simulink model "hcm_bicycle"  (R2017b)
settings: Solver=FixedStepAuto  StartTime=0.0  StopTime=10.0  RelTol=1e-3
values from neighbouring files (symbols this model uses):
  front_rear = 0    [init.m]
  setV = 0    [init.m]
  your_dut = 18    [init.m]
undefined symbols (not defined in the file or in its folder): hcm, sigbuilder_block, Zs0, Zu0
libraries: simulink x1
settings Model: Creator=rvorster  LastModifiedBy=rvorster

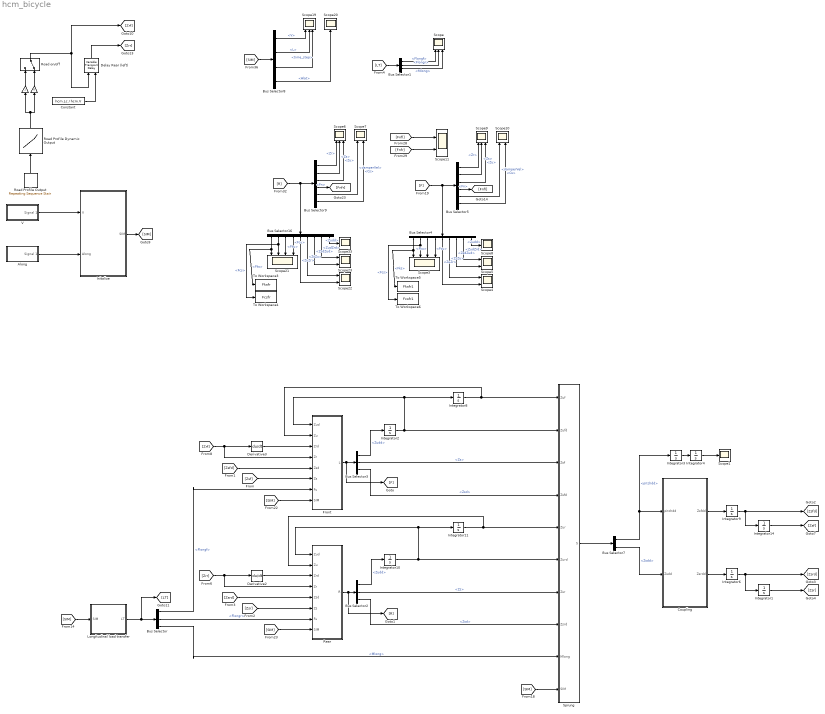
== system hcm_bicycle ==
  " " : Gain
  " " : Gain  Gain=0
  Along : Subsystem  Tag=STV Subsys  LoadFcn=sigbuilder_block('load');  StartFcn=sigbuilder_block('start');  StopFcn=sigbuilder_block('stop');  ClipboardFcn=sigbuilder_block('clipboard');  mask(Sigbuilder block){tuvar=[0:10]}
      mask help: Simulink:masks:SigbuilderBlock_MD
      mask init:
      | if ~strcmp(get_param(bdroot(gcbh),'SimulationStatus'),'stopped') tuvar = sigbuilder_block('maskInit'); end
      settings: CopyFcn=sigbuilder_block('copy');  DeleteFcn=sigbuilder_block('delete');  ModelCloseFcn=sigbuilder_block('modelClose');  PreSaveFcn=sigbuilder_block('preSave');  PauseFcn=sigbuilder_block('pause');  ContinueFcn=sigbuilder_block('continue');  NameChangeFcn=sigbuilder_block('namechange');  OpenFcn=sigbuilder_block('open',[429.75 192 565.5 402.75 ]);  CloseFcn=sigbuilder_block('close');
      mask Display: plot(0, 0, 100, 100,[2, 2, 32, 32, 2], [68, 8, 8, 68, 68],[32, 2], [38, 38], [32, 19, 2],[53, 60, 44], [32, 17, 17, 2],[16, 16, 31, 31]);txt = getActiveGroup(gcbh);text(2, 100, txt,'verticalAlignment', 'top');
  Bus Selector : BusSelector  OutputSignals=Flongf,Flongr,Mlong
  Bus Selector1 : BusSelector  OutputSignals=Flongf,Flongr,Mlong
  Bus Selector16 : BusSelector  OutputSignals=Fks,Fcs,Fku,Fcu,ZuZr,ZsZu,ZsdZud,ZudZrd,Zudd
  Bus Selector2 : BusSelector  OutputSignals=Zudd,Zs,Zsd
  Bus Selector3 : BusSelector  OutputSignals=Zudd,Zs,Zsd
  Bus Selector4 : BusSelector  OutputSignals=Fks,Fcs,Fku,Fcu,ZuZr,ZsZu,ZsdZud,ZudZrd,Zudd
  Bus Selector5 : BusSelector  OutputSignals=Zr,Zs,Zu,Fn,damperVel,Cs
  Bus Selector7 : BusSelector  OutputSignals=pitchdd,Zsdd
  Bus Selector8 : BusSelector  OutputSignals=V,L,time_step,Alat
  Bus Selector9 : BusSelector  OutputSignals=Zr,Zs,Zu,Fn,damperVel,Cs
  Constant : Constant  Value=hcm.Lc / hcm.V
  Coupling : MATLAB Function  TreatAsAtomicUnit=on
  Delay Rear (left) : VariableTransportDelay  VariableDelayType=Variable transport delay  MaximumDelay=10  MaximumPoints=4096
  Derivative2 : Derivative
  Derivative3 : Derivative
  Front : MATLAB Function  TreatAsAtomicUnit=on
  Initalize : MATLAB Function  TreatAsAtomicUnit=on
  Integrator1 : Integrator  InitialCondition=-Zs0(3)
  Integrator{2..4,6,9..10} (6 alike) : Integrator
  Integrator11 : Integrator  InitialCondition=-Zu0(3)
  Integrator14 : Integrator  InitialCondition=-Zs0(1)
  Integrator8 : Integrator  InitialCondition=-Zu0(1)
  Longitudinal load transfer : MATLAB Function  TreatAsAtomicUnit=on
  Rear : MATLAB Function  TreatAsAtomicUnit=on
  Road Profile Dynamic Output : Lookup_n-D  NumberOfTableDimensions=1  BreakpointsForDimension1=[-5:5]  Table=tanh([-5:5])  InternalRulePriority=Speed  RndMeth=Simplest  InputSameDT=on
  Road Profile Output : simulink/Sources/Repeating Sequence Stair  OutValues=hx_left  tsamp=time_step  OutMin=[]  OutMax=[]  OutDataTypeStr=double  OutputDataTypeScalingMode=double  OutDataType=fixdt(0,8)  ConRadixGroup=Best Precision: Vector-wise  OutScaling=2^-12
  "Road on/off " : ManualSwitch  CurrentSetting=0
  Scope{,6,9,19} (4 alike) : Scope  NumInputPorts=3
  Scope{1,8,20,33} (4 alike) : Scope
  Scope{4..5,7,10..11,22..23} (7 alike) : Scope  NumInputPorts=2
  Scope21 : Scope  NumInputPorts=4
  Scope3 : Scope  NumInputPorts=4
  Sprung : MATLAB Function  TreatAsAtomicUnit=on
  To Workspace3 : ToWorkspace  VariableName=Fksfr  SaveFormat=Timeseries  SampleTime=-1
  To Workspace4 : ToWorkspace  VariableName=Fcsfr  SaveFormat=Timeseries  SampleTime=-1
  To Workspace5 : ToWorkspace  VariableName=Fksfr1  SaveFormat=Timeseries  SampleTime=-1
  To Workspace6 : ToWorkspace  VariableName=Fcsfr1  SaveFormat=Timeseries  SampleTime=-1
  V : Subsystem  Tag=STV Subsys  LoadFcn=sigbuilder_block('load');  StartFcn=sigbuilder_block('start');  StopFcn=sigbuilder_block('stop');  ClipboardFcn=sigbuilder_block('clipboard');  mask(Sigbuilder block){tuvar=[0:10]}
      mask help: Simulink:masks:SigbuilderBlock_MD
      mask init:
      | if ~strcmp(get_param(bdroot(gcbh),'SimulationStatus'),'stopped') tuvar = sigbuilder_block('maskInit'); end
      settings: CopyFcn=sigbuilder_block('copy');  DeleteFcn=sigbuilder_block('delete');  ModelCloseFcn=sigbuilder_block('modelClose');  PreSaveFcn=sigbuilder_block('preSave');  PauseFcn=sigbuilder_block('pause');  ContinueFcn=sigbuilder_block('continue');  NameChangeFcn=sigbuilder_block('namechange');  OpenFcn=sigbuilder_block('open',[433.5 195.75 558 401.25 ]);  CloseFcn=sigbuilder_block('close');
      mask Display: plot(0, 0, 100, 100,[2, 2, 32, 32, 2], [68, 8, 8, 68, 68],[32, 2], [38, 38], [32, 19, 2],[53, 60, 44], [32, 17, 17, 2],[16, 16, 31, 31]);txt = getActiveGroup(gcbh);text(2, 100, txt,'verticalAlignment', 'top');
  wires:
  Integrator9/1 -> [Zsfd], Integrator14/1
  Bus Selector5/1 -> Scope9/1  "<Zr>"
  Bus Selector4/2 -> To Workspace6/1, Scope3/2  "<Fcs>"
  Coupling/2(Zsrdd) -> Integrator6/1
  Bus Selector9/2 -> Scope6/2  "<Zs>"
  [SIM] -> Rear/8(SIM)
  Bus Selector4/1 -> To Workspace5/1, Scope3/1  "<Fks>"
  Bus Selector2/1 -> Integrator10/1  "<Zudd>"
  Road Profile Output/1 -> Road Profile Dynamic Output/1
  [SIM] -> Bus Selector8/1
  Bus Selector9/4 -> [Fnfr]  "<Fn>"
  Bus Selector8/3 -> Scope19/3  "<time_step>"
  Constant/1 -> Delay Rear (left)/2
  [SIM] -> Front/8(SIM)
  Road Profile Dynamic Output/1 -> " "/1, " "/1
  Bus Selector4/8 -> Scope5/1  "<ZudZrd>"
  Integrator2/1 -> Sprung/2(Zufd), Front/1(Zud), Integrator8/1
  [SIM] -> Longitudinal load transfer/1(SIM)
  Delay Rear (left)/1 -> [Zrr]
  V/1(Signal 1) -> Initalize/1(V)
  Initalize/1(SIM) -> [SIM]
  Bus Selector8/1 -> Scope19/1  "<V>"
  Integrator1/1 -> [Zsr]
  Front/1(L) -> [F], Bus Selector3/1
  [Zrr] -> Rear/4(Zr), Derivative2/1
  Bus Selector8/4 -> Scope20/1  "<Alat>"
  Bus Selector9/1 -> Scope6/1  "<Zr>"
  Coupling/1(Zsfdd) -> Integrator9/1
  Bus Selector4/6 -> Scope4/1  "<ZsZu>"
  [F] -> Bus Selector5/1, Bus Selector4/1
  [Fnfr] -> Scope11/2
  Bus Selector4/4 -> Scope3/4  "<Fcu>"
  Bus Selector5/3 -> Scope9/3  "<Zu>"
  Bus Selector5/2 -> Scope9/2  "<Zs>"
  Bus Selector3/1 -> Integrator2/1  "<Zudd>"
  Bus Selector16/3 -> Scope21/3  "<Fku>"
  Bus Selector3/3 -> Sprung/4(Zsfd)  "<Zsd>"
  Bus Selector16/5 -> Scope22/2  "<ZuZr>"
  Bus Selector16/4 -> Scope21/4  "<Fcu>"
  Bus Selector5/6 -> Scope10/2  "<Cs>"
  Bus Selector16/6 -> Scope22/1  "<ZsZu>"
  Bus Selector4/7 -> Scope5/2  "<ZsdZud>"
  Bus Selector/2 -> Rear/7(Fu)  "<Flongr>"
  Along/1(Signal 1) -> Initalize/2(Along)
  [R] -> Bus Selector9/1, Bus Selector16/1
  Bus Selector9/3 -> Scope6/3  "<Zu>"
  Integrator8/1 -> Front/2(Zu), Sprung/1(Zuf)
  Bus Selector16/7 -> Scope23/2  "<ZsdZud>"
  Rear/1(R) -> [R], Bus Selector2/1
  Bus Selector5/4 -> [Fnfl]  "<Fn>"
  Derivative2/1 -> Rear/3(Zrd)
  Bus Selector16/8 -> Scope23/1  "<ZudZrd>"
  Integrator6/1 -> [Zsrd], Integrator1/1
  "Road on/off "/1 -> [Zrf], Delay Rear (left)/1
  Bus Selector7/2 -> Coupling/2(Zsdd)  "<Zsdd>"
  Bus Selector9/5 -> Scope7/1  "<damperVel>"
  Bus Selector2/2 -> Sprung/7(Zsr)  "<Zs>"
  Bus Selector5/5 -> Scope10/1  "<damperVel>"
  [Zsfd] -> Front/5(Zsd)
  Bus Selector2/3 -> Sprung/8(Zsrd)  "<Zsd>"
  Sprung/1(S) -> Bus Selector7/1
  Bus Selector8/2 -> Scope19/2  "<L>"
  Bus Selector16/9 -> Scope33/1  "<Zudd>"
  Bus Selector4/3 -> Scope3/3  "<Fku>"
  " "/1 -> "Road on/off "/2
  [Zsr] -> Rear/6(Zs)
  Bus Selector4/9 -> Scope8/1  "<Zudd>"
  Bus Selector16/2 -> To Workspace4/1, Scope21/2  "<Fcs>"
  Integrator14/1 -> [Zsf]
  " "/1 -> "Road on/off "/1
  [LT] -> Bus Selector1/1
  Bus Selector3/2 -> Sprung/3(Zsf)  "<Zs>"
  Bus Selector9/6 -> Scope7/2  "<Cs>"
  Derivative3/1 -> Front/3(Zrd)
  [SIM] -> Sprung/10(SIM)
  [Fnfl] -> Scope11/1
  [Zsrd] -> Rear/5(Zsd)
  [Zsf] -> Front/6(Zs)
  Bus Selector16/1 -> To Workspace3/1, Scope21/1  "<Fks>"
  Integrator11/1 -> Rear/2(Zu), Sprung/5(Zur)
  Bus Selector4/5 -> Scope4/2  "<ZuZr>"
  Bus Selector/1 -> Front/7(Fu)  "<Flongf>"
  [Zrf] -> Front/4(Zr), Derivative3/1
  Longitudinal load transfer/1(LT) -> [LT], Bus Selector/1
  Integrator10/1 -> Rear/1(Zud), Integrator11/1, Sprung/6(Zurd)
  Bus Selector/3 -> Sprung/9(Mlong)  "<Mlong>"
  Bus Selector1/1 -> Scope/1  "<Flongf>"
  Bus Selector1/2 -> Scope/2  "<Flongr>"
  Bus Selector1/3 -> Scope/3  "<Mlong>"
  Bus Selector7/1 -> Coupling/1(pitchdd), Integrator3/1  "<pitchdd>"
  Integrator3/1 -> Integrator4/1
  Integrator4/1 -> Scope1/1

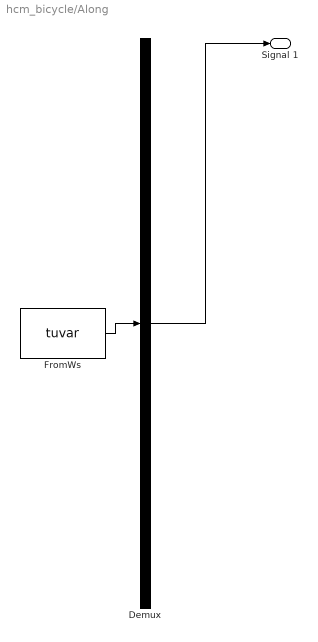
== system hcm_bicycle/Along ==
  Demux : Demux  Tag=STV Demux  Outputs=1
  FromWs : FromWorkspace  Tag=STV FromWs  VariableName=tuvar  SampleTime=0
      SigBuilderData=|
      | common.afterFinalStr = 'Extrapolate'
      | common.sampleTime = 0
      | dataSet.timeRange = [0 10]
      | dataSet.name = 'Group 1'
      | sbobj.Groups.Name = 'Group 1'
      | sbobj.Groups.Signals.Name = 'Signal 1'
      | sbobj.Groups.Signals.XData = [0 4 6 10]
      | sbobj.Groups.Signals.YData = [0 0 0 0]
  Signal 1 : Outport  Tag=STV Outport
  wires:
  Demux/1 -> Signal 1/1
  FromWs/1 -> Demux/1

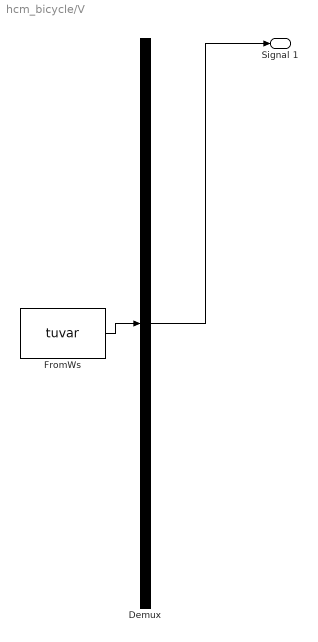
== system hcm_bicycle/V ==
  Demux : Demux  Tag=STV Demux  Outputs=1
  FromWs : FromWorkspace  Tag=STV FromWs  VariableName=tuvar  SampleTime=0
      SigBuilderData=|
      | common.afterFinalStr = 'Extrapolate'
      | common.sampleTime = 0
      | dataSet.timeRange = [0 10]
      | dataSet.name = 'Group 1'
      | sbobj.Groups.Name = 'Group 1'
      | sbobj.Groups.Signals.Name = 'Signal 1'
      | sbobj.Groups.Signals.XData = [0 4 6 10]
      | sbobj.Groups.Signals.YData = [0 35 0 0]
  Signal 1 : Outport  Tag=STV Outport
  wires:
  Demux/1 -> Signal 1/1
  FromWs/1 -> Demux/1

== matlab function hcm_bicycle/Rear ==
  data: Zud input; Zu input; Zrd input; Zr input; Zsd input; Zs input; Fu input; hcm parameter; R output Bus: U; SIM input Bus: SIM; Zs0 parameter
function R = fcn(Zud, Zu, Zrd, Zr, Zsd, Zs, Fu, hcm, SIM, Zs0)
    
    loc = 3;
    R = unsprung_mass(Zud, Zu, Zrd, Zr, Zsd, Zs, Fu, loc, SIM, Zs0, hcm);

end

== matlab function hcm_bicycle/Front ==
  data: Zud input; Zu input; Zrd input; Zr input; Zsd input; Zs input; Fu input; hcm parameter; L output Bus: U; SIM input Bus: SIM; Zs0 parameter
function L = fcn(Zud, Zu, Zrd, Zr, Zsd, Zs, Fu, hcm, SIM, Zs0)
    
    loc = 1;
    L = unsprung_mass(Zud, Zu, Zrd, Zr, Zsd, Zs, Fu, loc, SIM, Zs0, hcm);

end

== matlab function hcm_bicycle/Sprung ==
  data: Zuf input; Zufd input; S output Bus: C; Zsf input; Zsfd input; Zur input; Zurd input; Zsr input; Zsrd input; Mlong input; SIM input Bus: SIM; hcm parameter
function S = fcn(Zuf, Zufd, Zsf, Zsfd, Zur, Zurd, Zsr, Zsrd, Mlong, SIM, hcm)   
    
    S = sprung_mass_bicycle(Zuf, Zufd, Zsf, Zsfd, Zur, Zurd, Zsr, ... 
        Zsrd, Mlong, SIM, hcm);

end

== matlab function hcm_bicycle/Longitudinal load transfer ==
  data: LT output Bus: LT; hcm parameter; SIM input Bus: SIM
function LT = fcn(hcm, SIM)
    
    [Flongf, Flongr, Mlong] = longitudinal_load(SIM, hcm);
    
    LT.Flat = 0;
    LT.Mlat = 0;
    LT.Flongf = Flongf;
    LT.Flongr = Flongr;
    LT.Mlong = Mlong;
    LT.Ful = 0;
    LT.Fur = 0;
    
end

== matlab function hcm_bicycle/Coupling ==
  data: pitchdd input; Zsfdd output; Zsrdd output; Zsdd input; hcm parameter
function [Zsfdd, Zsrdd] = fcn(pitchdd, Zsdd, hcm)

    [Zsfdd, Zsrdd] = coupling_bicycle(Zsdd, pitchdd, hcm);

end

== matlab function hcm_bicycle/Initalize ==
  settings: updateMethod=DISCRETE
  data: V input; Along input; hcm parameter; SIM output Bus: SIM; setV parameter; front_rear parameter; your_dut parameter
function SIM = fcn(V, Along, hcm, setV, front_rear, your_dut)

    if (setV == 0)
        SIM.V = hcm.V;
        SIM.L = 0.5*hcm.V^2*hcm.ClA*hcm.rho0;
        SIM.Alat = 0;
        SIM.Along = hcm.Along;
        SIM.sim_time = 0;
        SIM.sim_step = 0;
        SIM.time_step = 0.01 / hcm.V;
        SIM.your_dut = your_dut;
        SIM.front_rear = front_rear;
    else
        SIM.V = V;
        SIM.L = 0.5*V^2*hcm.ClA*hcm.rho0;
        SIM.Alat = 0;
        SIM.Along = Along;
        SIM.sim_time = 0;
        SIM.sim_step = 0;
        SIM.time_step = 0.01 / V;
        SIM.your_dut = your_dut;
        SIM.front_rear = front_rear;
    end

end
